simulink model "Backstepping"  (R2022b)
settings: Solver=ode4  StartTime=0.0  StopTime=tsamplesimulink  FixedStep=0.001  RelTol=1e-3
undefined symbols (not defined in the file): Ac, Bcg, Cc, Dcg, Lambda1, Lambda2, N, tm, v1, v2, v3, v4
settings Model: Creator=Isaac  LastModifiedBy=mgotor
settings SolverCC: AlgebraicLoopSolver=TrustRegion
settings DataIOCC: ReturnWorkspaceOutputs=off
settings DebuggingCC: UnconnectedInputMsg=warning  UnconnectedOutputMsg=warning  UnconnectedLineMsg=warning  ArithmeticOperatorsInVariantConditions=warning
settings ModelReferenceCC: EnableRefExpFcnMdlSchedulingChecks=on
settings SFSimCC: SimUseLocalCustomCode=off  CustomCodeUndefinedFunction=UseInterfaceOnly
settings RTWCC: RTWUseLocalCustomCode=off
settings CodeAppCC: StateflowObjectComments=on

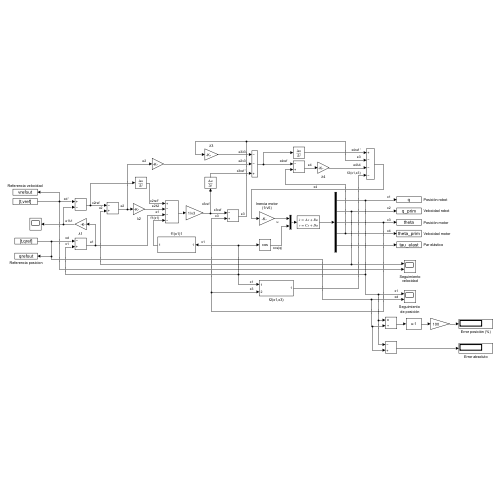
[thumbnail: Simulink's stored preview of the top-level diagram]
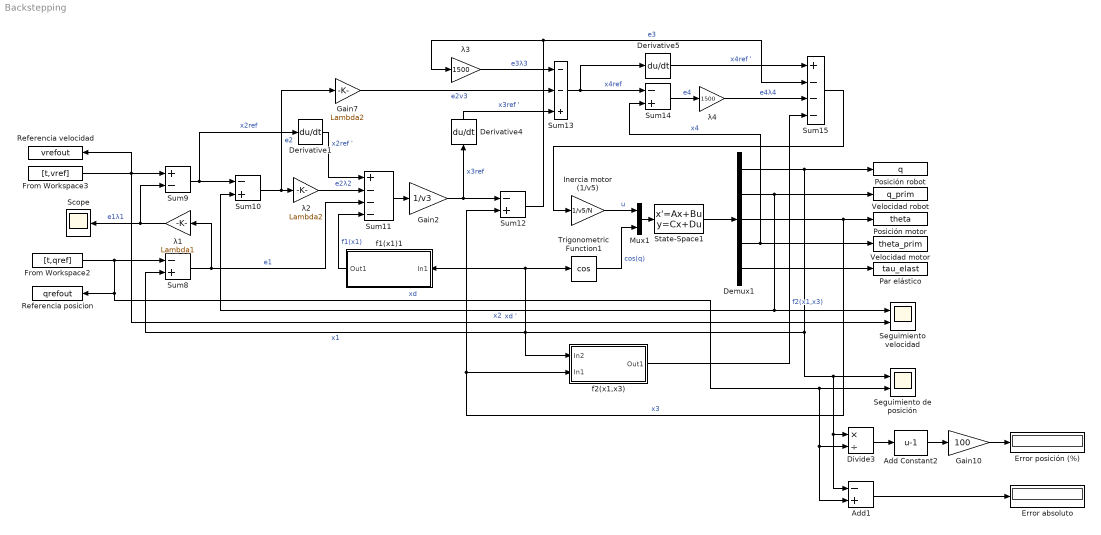
== system Backstepping ==
  Add Constant2 : Bias  Bias=-1  SaturateOnIntegerOverflow=off
  Add1 : Sum  Inputs=-+
  Demux1 : Demux  Outputs=5
  Derivative1 : Derivative
  Derivative4 : Derivative
  Derivative5 : Derivative
  Divide3 : Product  Inputs=*/
  Error absoluto : Display
  Error posición (%) : Display
  From Workspace2 : FromWorkspace  VariableName=[t,qref]  SampleTime=tm  ZeroCross=off
  From Workspace3 : FromWorkspace  VariableName=[t,vref]  SampleTime=tm  ZeroCross=off
  Gain10 : Gain  Gain=100
  Gain2 : Gain  Gain=1/v3
  Gain7 : Gain  Gain=Lambda2
  Inercia motor (1/v5) : Gain  Gain=1/v5/N  SaturateOnIntegerOverflow=on  OutDataTypeStr=Inherit: Same as input  ParamDataTypeStr=Inherit: Same as input
  Mux1 : Mux  Inputs=2
  Par elástico : ToWorkspace  VariableName=tau_elast  SaveFormat=Timeseries  SampleTime=tm
  Posición motor : ToWorkspace  VariableName=theta  SaveFormat=Timeseries  SampleTime=tm
  Posición robot : ToWorkspace  VariableName=q  SaveFormat=Timeseries  SampleTime=tm
  Referencia posicion : ToWorkspace  VariableName=qrefout  SaveFormat=Timeseries  SampleTime=tm
  Referencia velocidad : ToWorkspace  VariableName=vrefout  SaveFormat=Timeseries  SampleTime=tm
  Scope : Scope
  Seguimiento velocidad : Scope  NumInputPorts=2
  Seguimiento de posición : Scope  NumInputPorts=2
  State-Space1 : StateSpace  A=Ac  B=Bcg  C=Cc  D=Dcg  InitialCondition=0  ParameterTunability=Unconstrained
  Sum{8,10,12,14} (4 alike) : Sum  Inputs=-+
  Sum11 : Sum  Inputs=+---
  Sum13 : Sum  Inputs=--+
  Sum15 : Sum  Inputs=+---
  Sum9 : Sum  Inputs=+-
  Trigonometric Function1 : Trigonometry  Operator=cos
  Velocidad motor : ToWorkspace  VariableName=theta_prim  SaveFormat=Timeseries  SampleTime=tm
  Velocidad robot : ToWorkspace  VariableName=q_prim  SaveFormat=Timeseries  SampleTime=tm
  f1(x1)1 : Subsystem
  f2(x1,x3) : Subsystem
  λ1 : Gain  Gain=Lambda1
  λ2 : Gain  Gain=Lambda2
  λ3 : Gain  Gain=1500
  λ4 : Gain  Gain=1500
  wires:
  Gain7/1 -> Sum13/2  "e2v3"
  Divide3/1 -> Add Constant2/1
  Mux1/1 -> State-Space1/1
  From Workspace2/1 -> Sum8/1, Referencia posicion/1, Add1/2, Divide3/2, Seguimiento de posición/2  "xd"
  Sum15/1 -> Inercia motor (1/v5)/1
  λ1/1 -> Sum9/2, Scope/1  "e1λ1"
  Sum14/1 -> λ4/1  "e4"
  Gain10/1 -> Error posición (%)/1
  Demux1/5 -> Par elástico/1
  Sum12/1 -> λ3/1, Sum15/2  "e3"
  Add1/1 -> Error absoluto/1
  Add Constant2/1 -> Gain10/1
  Demux1/4 -> Sum14/2, Velocidad motor/1  "x4"
  Derivative5/1 -> Sum15/1  "x4ref '"
  Demux1/2 -> Seguimiento velocidad/1, Sum10/2, Velocidad robot/1  "x2"
  Derivative4/1 -> Sum13/3  "x3ref '"
  Sum10/1 -> Gain7/1, λ2/1  "e2"
  Sum8/1 -> λ1/1, Sum11/3  "e1"
  λ2/1 -> Sum11/2  "e2λ2"
  f1(x1)1/1(Out1) -> Sum11/4  "f1(x1)"
  Gain2/1 -> Derivative4/1, Sum12/1  "x3ref"
  f2(x1,x3)/1(Out1) -> Sum15/4  "f2(x1,x3)"
  λ3/1 -> Sum13/1  "e3λ3"
  Derivative1/1 -> Sum11/1  "x2ref '"
  Sum11/1 -> Gain2/1
  From Workspace3/1 -> Referencia velocidad/1, Sum9/1, Seguimiento velocidad/2  "xd '"
  Sum9/1 -> Sum10/1, Derivative1/1  "x2ref"
  State-Space1/1 -> Demux1/1
  Demux1/1 -> Sum8/2, f2(x1,x3)/1(In2), f1(x1)1/1(In1), Trigonometric Function1/1, Seguimiento de posición/1, Add1/1, Divide3/1, Posición robot/1  "x1"
  Demux1/3 -> Posición motor/1, Sum12/2, f2(x1,x3)/2(In1)  "x3"
  Inercia motor (1/v5)/1 -> Mux1/1  "u"
  Trigonometric Function1/1 -> Mux1/2  "cos(q)"
  λ4/1 -> Sum15/3  "e4λ4"
  Sum13/1 -> Derivative5/1, Sum14/1  "x4ref"

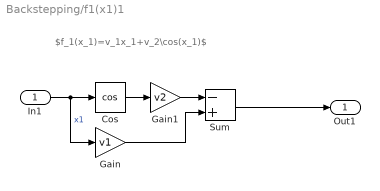
== system Backstepping/f1(x1)1 ==
  note: $f_1(x_1)=v_1x_1+v_2\cos(x_1)$
  In1 : Inport
  Cos : Trigonometry  Operator=cos
  Gain : Gain  Gain=v1
  Gain1 : Gain  Gain=v2
  Sum : Sum  Inputs=-+
  Out1 : Outport
  wires:
  Cos/1 -> Gain1/1
  Gain/1 -> Sum/2
  In1/1 -> Gain/1, Cos/1  "x1"
  Sum/1 -> Out1/1
  Gain1/1 -> Sum/1

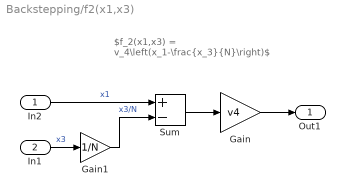
== system Backstepping/f2(x1,x3) ==
  note: $f_2(x1,x3) = v_4\left(x_1-\frac{x_3}{N}\right)$
  In2 : Inport
  In1 : Inport  Port=2
  Gain : Gain  Gain=v4
  Gain1 : Gain  Gain=1/N
  Sum : Sum  Inputs=+-
  Out1 : Outport
  wires:
  In2/1 -> Sum/1  "x1"
  Sum/1 -> Gain/1
  Gain/1 -> Out1/1
  In1/1 -> Gain1/1  "x3"
  Gain1/1 -> Sum/2  "x3/N"
